simulink model "Ref42_SFPPC_compare"  (R2025b)
settings: Solver=ode4  StartTime=0.0  StopTime=20  FixedStep=0.001  RelTol=1e-3
settings Model: Creator=31586  LastModifiedBy=31586

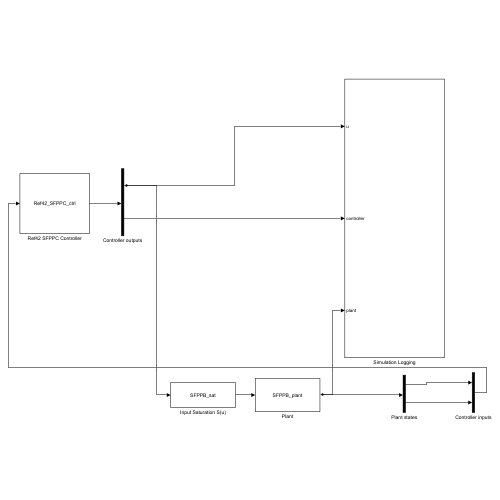
[thumbnail: Simulink's stored preview of the top-level diagram]
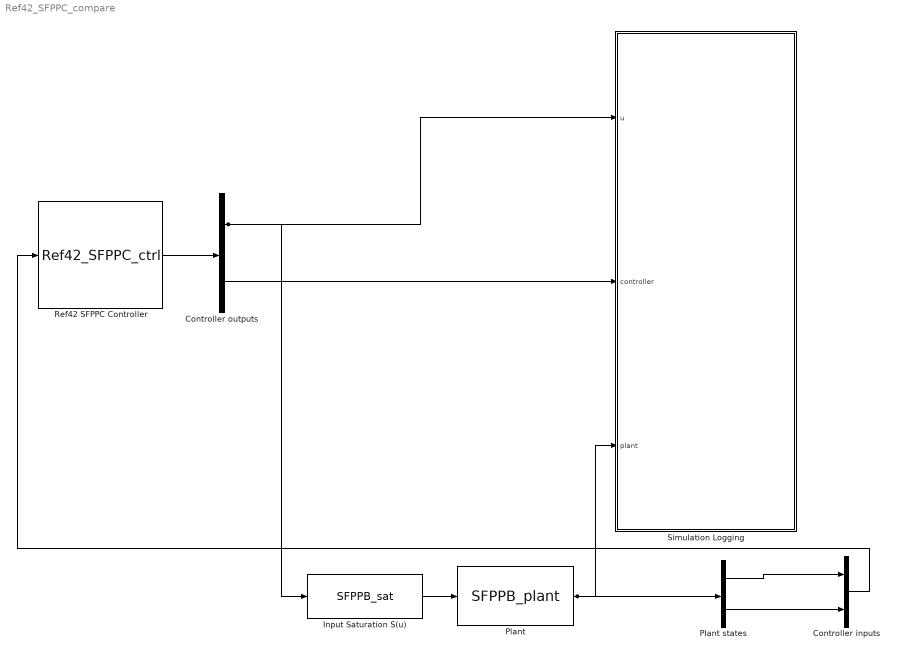
== system Ref42_SFPPC_compare ==
  Controller inputs : Mux  Inputs=2
  Controller outputs : Demux  Outputs=[1 12]
  Input Saturation S(u) : S-Function  Description=Eq. (2): S(u) = sgn(u)*u_d if |u|>u_d  FunctionName=SFPPB_sat  SFunctionDeploymentMode=off  EnableBusSupport=off
  Plant : S-Function  FunctionName=SFPPB_plant  SFunctionDeploymentMode=off  EnableBusSupport=off
  Plant states : Demux  Outputs=2
  Ref42 SFPPC Controller : S-Function  Description=Reference [42] SFPPC: Eqs. (24)-(25),(33),(39)-(40)  FunctionName=Ref42_SFPPC_ctrl  SFunctionDeploymentMode=off  EnableBusSupport=off
  Simulation Logging : Subsystem
  wires:
  Controller outputs/2 -> Simulation Logging/2(controller)
  Controller outputs/1 -> Input Saturation S(u)/1, Simulation Logging/1(u)
  Ref42 SFPPC Controller/1 -> Controller outputs/1
  Input Saturation S(u)/1 -> Plant/1
  Plant states/2 -> Controller inputs/2
  Plant/1 -> Plant states/1, Simulation Logging/3(plant)
  Plant states/1 -> Controller inputs/1
  Controller inputs/1 -> Ref42 SFPPC Controller/1

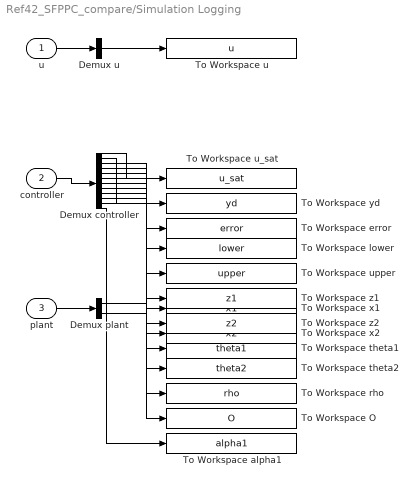
== system Ref42_SFPPC_compare/Simulation Logging ==
  u : Inport
  controller : Inport  Port=2
  plant : Inport  Port=3
  Demux controller : Demux  Outputs=12
  Demux plant : Demux  Outputs=2
  Demux u : Demux  Outputs=1
  To Workspace O : ToWorkspace  VariableName=O  SaveFormat=Timeseries  SampleTime=-1
  To Workspace alpha1 : ToWorkspace  VariableName=alpha1  SaveFormat=Timeseries  SampleTime=-1
  To Workspace error : ToWorkspace  VariableName=error  SaveFormat=Timeseries  SampleTime=-1
  To Workspace lower : ToWorkspace  VariableName=lower  SaveFormat=Timeseries  SampleTime=-1
  To Workspace rho : ToWorkspace  VariableName=rho  SaveFormat=Timeseries  SampleTime=-1
  To Workspace theta1 : ToWorkspace  VariableName=theta1  SaveFormat=Timeseries  SampleTime=-1
  To Workspace theta2 : ToWorkspace  VariableName=theta2  SaveFormat=Timeseries  SampleTime=-1
  To Workspace u : ToWorkspace  VariableName=u  SaveFormat=Timeseries  SampleTime=-1
  To Workspace u_sat : ToWorkspace  VariableName=u_sat  SaveFormat=Timeseries  SampleTime=-1
  To Workspace upper : ToWorkspace  VariableName=upper  SaveFormat=Timeseries  SampleTime=-1
  To Workspace x1 : ToWorkspace  VariableName=x1  SaveFormat=Timeseries  SampleTime=-1
  To Workspace x2 : ToWorkspace  VariableName=x2  SaveFormat=Timeseries  SampleTime=-1
  To Workspace yd : ToWorkspace  VariableName=yd  SaveFormat=Timeseries  SampleTime=-1
  To Workspace z1 : ToWorkspace  VariableName=z1  SaveFormat=Timeseries  SampleTime=-1
  To Workspace z2 : ToWorkspace  VariableName=z2  SaveFormat=Timeseries  SampleTime=-1
  wires:
  ? -> ?
  u/1 -> Demux u/1
  Demux u/1 -> To Workspace u/1
  controller/1 -> Demux controller/1
  Demux controller/1 -> To Workspace u_sat/1
  Demux controller/2 -> To Workspace yd/1
  Demux controller/3 -> To Workspace error/1
  Demux controller/4 -> To Workspace lower/1
  Demux controller/5 -> To Workspace upper/1
  Demux controller/6 -> To Workspace z1/1
  Demux controller/7 -> To Workspace z2/1
  Demux controller/8 -> To Workspace theta1/1
  Demux controller/9 -> To Workspace theta2/1
  Demux controller/10 -> To Workspace rho/1
  Demux controller/11 -> To Workspace O/1
  Demux controller/12 -> To Workspace alpha1/1
  plant/1 -> Demux plant/1
  Demux plant/1 -> To Workspace x1/1
  Demux plant/2 -> To Workspace x2/1
